simulink subsystem "AS_Blower"  (R2022b)
settings: Solver=VariableStepAuto  StartTime=0.0  StopTime=10.0  RelTol=1e-3
undefined symbols (not defined in the file): BlowerMaxFlow
libraries: nesl_utility x1, fl_lib x1
settings Model: DefaultTestHarness=AS_Blower_Harness1  Creator=CSN-Simulation  LastModifiedBy=MATLAB
settings DebuggingCC: UnconnectedInputMsg=warning  UnconnectedOutputMsg=warning  UnconnectedLineMsg=warning
settings ModelReferenceCC: EnableRefExpFcnMdlSchedulingChecks=on
settings RTWCC: DLArmComputeVersion=19.05

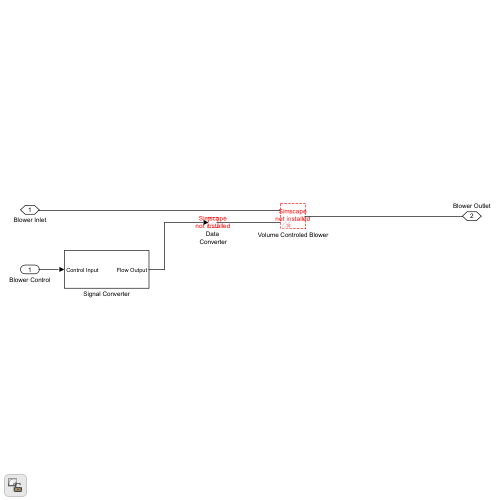
[thumbnail: Simulink's stored preview of the top-level diagram]
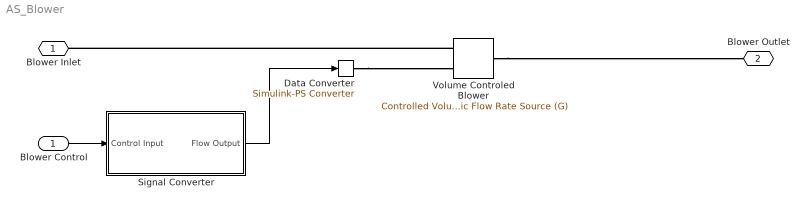
== system AS_Blower ==
  Blower Control : Inport
  Data Converter : nesl_utility/Simulink-PS Converter  PhysicalDomain=network_engine_domain  SubClassName=ps_input  LeftPortType=input  RightPortType=output  PseudoPeriodic=off  Frequencies=[]  NoiseDistribution=none  NoiseParameters=[]  Unit=m^3/s  AffineConversion=off  FilteringAndDerivatives=provide  SimscapeFilterOrder=1  InputFilterTimeConstant=0.001  UdotUserProvided=0
  Signal Converter : Subsystem
  Volume Controled Blower : fl_lib/Gas/Sources/Controlled Volumetric Flow Rate Source (G)  power_spec=foundation.enum.power_spec.none  area_A=106.81 mm^2  area_B=94.25 mm^2
      settings: InternalSimscapePortConfiguration="{\"Bottom\":[],\"Left\":[{\"id\":\"A\",\"label\":\"A\",\"type\":\"foundation.gas.gas\"},{\"id\":\"V\",\"label\":\"V\",\"type\":\"input\"}],\"Right\":[{\"id\":\"B\",\"label\":\"B\",\"type\":\"foundation.gas.gas\"}],\"Top\":[]}"
  Blower Inlet : PMIOPort  Side=Left
  Blower Outlet : PMIOPort  Port=2  Side=Right
  wires:
  Blower Control/1 -> Signal Converter/1(Control Input)
  Signal Converter/1(Flow Output) -> Data Converter/1
  connections:
  Data Converter/RConn1 -- Volume Controled Blower/LConn2
  Volume Controled Blower/LConn1 -- Blower Inlet/RConn1
  Volume Controled Blower/RConn1 -- Blower Outlet/RConn1

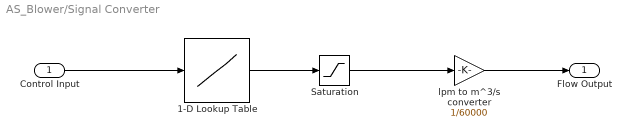
== system AS_Blower/Signal Converter ==
  Control Input : Inport
  1-D Lookup Table : Lookup_n-D  NumberOfTableDimensions=1  BreakpointsForDimension1=[0,1]  Table=[1,BlowerMaxFlow]  InternalRulePriority=Speed  RndMeth=Simplest
  Saturation : Saturate  UpperLimit=BlowerMaxFlow  LowerLimit=0
  lpm to m^3/s converter : Gain  Gain=1/60000
  Flow Output : Outport
  wires:
  Control Input/1 -> 1-D Lookup Table/1
  1-D Lookup Table/1 -> Saturation/1
  lpm to m^3/s converter/1 -> Flow Output/1
  Saturation/1 -> lpm to m^3/s converter/1
